simulink model "gm_CLKDIV_LED_basic"  (R2023a)
settings: Solver=VariableStepAuto  StartTime=0.0  StopTime=2  RelTol=1e-3
libraries: simulink x4
settings Model: Creator=criedl  LastModifiedBy=eduyilmet001
settings OptimizationCC: BlockReduction=off  ConditionallyExecuteInputs=off
settings DebuggingCC: ArtificialAlgebraicLoopMsg=none  InheritedTsInSrcMsg=none  UnconnectedInputMsg=warning  UnconnectedOutputMsg=warning  UnconnectedLineMsg=warning
settings ModelReferenceCC: EnableRefExpFcnMdlSchedulingChecks=on
settings RTWCC: DLArmComputeVersion=19.05

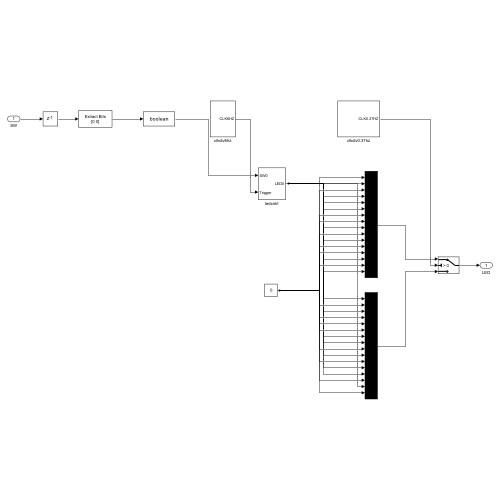
[thumbnail: Simulink's stored preview of the top-level diagram]
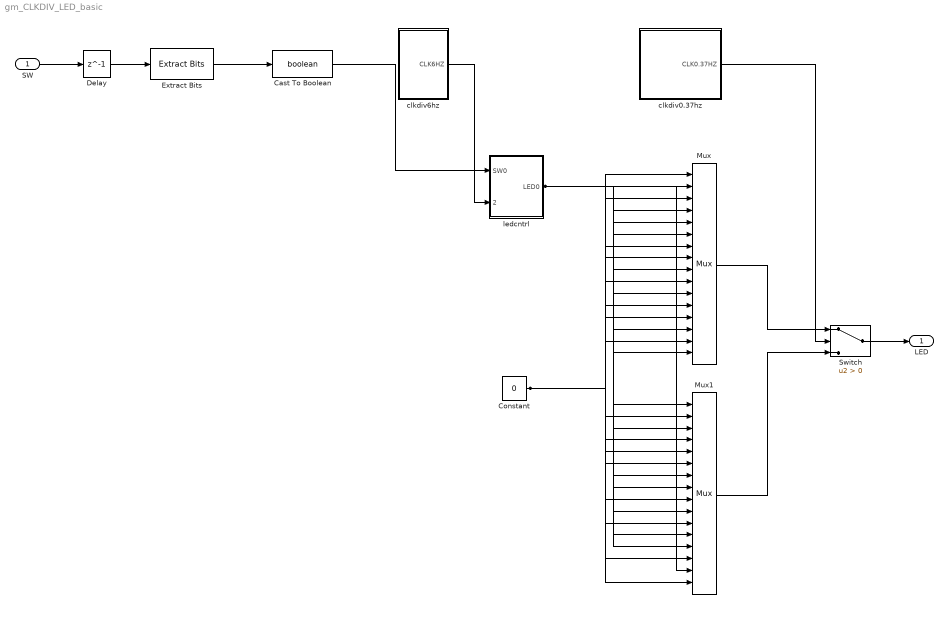
== system gm_CLKDIV_LED_basic ==
  SW : Inport  OutDataTypeStr=uint16  PortDimensions=1  SampleTime=1e-08
  Cast To Boolean : DataTypeConversion  OutDataTypeStr=boolean  SaturateOnIntegerOverflow=off  RndMeth=Floor
  Constant : Constant  Value=0  OutDataTypeStr=boolean
  Delay : Delay  DelayLength=1  InitialCondition=0
  Extract Bits : simulink/Logic and Bit Operations/Extract Bits  bitsToExtract=Range of bits  numBits=8  bitIdxRange=[0 0]  outScalingMode=Preserve fixed-point scaling
  Mux : Mux  Inputs=16
  Mux1 : Mux  Inputs=16
  Switch : Switch  Criteria=u2 > Threshold  SaturateOnIntegerOverflow=off  InputSameDT=off
  clkdiv0.37hz : Subsystem
  clkdiv6hz : Subsystem
  ledcntrl : Subsystem
  LED : Outport  SampleTime=1e-08  InitialOutput=0
  wires:
  SW/1 -> Delay/1
  Cast To Boolean/1 -> ledcntrl/1(SW0)
  Constant/1 -> Mux1/16, Mux1/14, Mux1/11, Mux1/9, Mux1/6, Mux1/5, Mux1/4, Mux1/2, Mux/15, Mux/13, Mux/12, Mux/10, Mux/8, Mux/7, Mux/3, Mux/1
  Delay/1 -> Extract Bits/1
  Extract Bits/1 -> Cast To Boolean/1
  Mux/1 -> Switch/1
  Mux1/1 -> Switch/3
  Switch/1 -> LED/1
  clkdiv0.37hz/1(CLK0.37HZ) -> Switch/2
  clkdiv6hz/1(CLK6HZ) -> ledcntrl/2(Trigger)
  ledcntrl/1(LED0) -> Mux1/15, Mux1/13, Mux1/12, Mux1/10, Mux1/8, Mux1/7, Mux1/3, Mux1/1, Mux/16, Mux/14, Mux/11, Mux/9, Mux/6, Mux/5, Mux/4, Mux/2

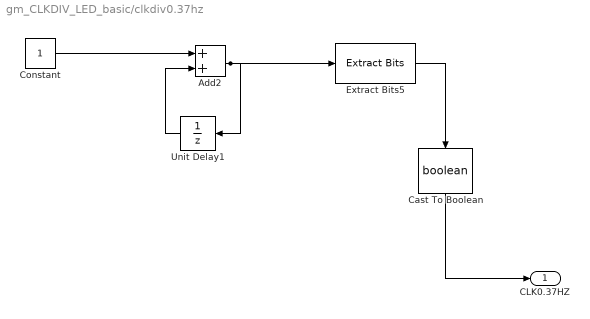
== system gm_CLKDIV_LED_basic/clkdiv0.37hz ==
  Add2 : Sum  AccumDataTypeStr=fixdt(0,29,0)  OutDataTypeStr=fixdt(0,29,0)
  Cast To Boolean : DataTypeConversion  OutDataTypeStr=boolean  SaturateOnIntegerOverflow=off  RndMeth=Floor
  Constant : Constant  OutDataTypeStr=boolean
  Extract Bits5 : simulink/Logic and Bit Operations/Extract Bits  bitsToExtract=Range of bits  numBits=8  bitIdxRange=[28 28]  outScalingMode=Preserve fixed-point scaling
  Unit Delay1 : UnitDelay  SampleTime=-1  HasFrameUpgradeWarning=on
  CLK0.37HZ : Outport  OutDataTypeStr=boolean  SampleTime=1e-08  InitialOutput=0
  wires:
  Add2/1 -> Extract Bits5/1, Unit Delay1/1
  Cast To Boolean/1 -> CLK0.37HZ/1
  Constant/1 -> Add2/1
  Extract Bits5/1 -> Cast To Boolean/1
  Unit Delay1/1 -> Add2/2

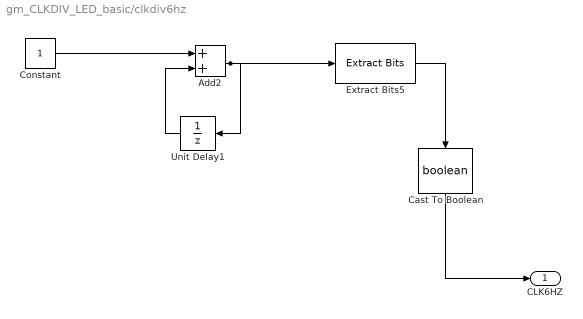
== system gm_CLKDIV_LED_basic/clkdiv6hz ==
  Add2 : Sum  AccumDataTypeStr=fixdt(0,24,0)  OutDataTypeStr=fixdt(0,24,0)
  Cast To Boolean : DataTypeConversion  OutDataTypeStr=boolean  SaturateOnIntegerOverflow=off  RndMeth=Floor
  Constant : Constant  OutDataTypeStr=boolean
  Extract Bits5 : simulink/Logic and Bit Operations/Extract Bits  bitsToExtract=Range of bits  numBits=8  bitIdxRange=[23 23]  outScalingMode=Preserve fixed-point scaling
  Unit Delay1 : UnitDelay  SampleTime=-1  HasFrameUpgradeWarning=on
  CLK6HZ : Outport  OutDataTypeStr=boolean  SampleTime=1e-08  InitialOutput=0
  wires:
  Add2/1 -> Extract Bits5/1, Unit Delay1/1
  Cast To Boolean/1 -> CLK6HZ/1
  Constant/1 -> Add2/1
  Extract Bits5/1 -> Cast To Boolean/1
  Unit Delay1/1 -> Add2/2

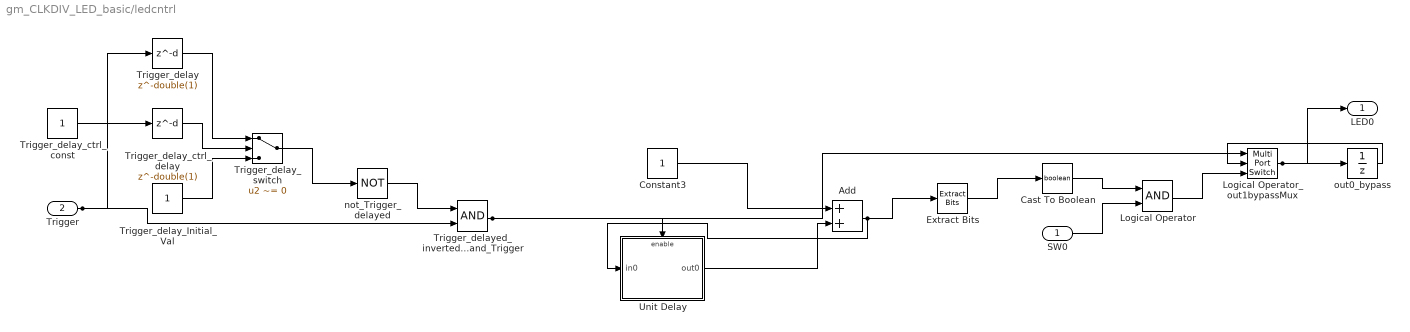
== system gm_CLKDIV_LED_basic/ledcntrl ==
  SW0 : Inport  OutDataTypeStr=boolean  PortDimensions=1  SampleTime=1e-08
  Trigger : Inport  Port=2  OutDataTypeStr=boolean  SampleTime=1e-08
  Add : Sum  AccumDataTypeStr=fixdt(0, 1, 0)  OutDataTypeStr=fixdt(0, 1, 0)  SampleTime=1e-08
  Cast To Boolean : DataTypeConversion  OutDataTypeStr=boolean  SampleTime=1e-08  SaturateOnIntegerOverflow=off  RndMeth=Floor
  Constant3 : Constant  OutDataTypeStr=boolean  SampleTime=1e-08
  Extract Bits : simulink/Logic and Bit Operations/Extract Bits  bitsToExtract=Range of bits  numBits=8  bitIdxRange=[0 0]  outScalingMode=Preserve fixed-point scaling
  Logical Operator : Logic  AllPortsSameDT=off  OutDataTypeStr=boolean  SampleTime=1e-08
  Logical Operator_out1bypassMux : MultiPortSwitch  DataPortOrder=Zero-based contiguous  Inputs=2  zeroidx=on  SampleTime=1e-08  SaturateOnIntegerOverflow=off  InputSameDT=off
  Trigger_delay : Delay  DelayLength=double(1)  InitialCondition=0
  Trigger_delay_Initial_Val : Constant  OutDataTypeStr=boolean  SampleTime=1e-08
  Trigger_delay_ctrl_const : Constant  OutDataTypeStr=boolean  SampleTime=1e-08
  Trigger_delay_ctrl_delay : Delay  DelayLength=double(1)  InitialCondition=0
  Trigger_delay_switch : Switch  Criteria=u2 ~= 0  Threshold=double(0)  OutDataTypeStr=boolean  SampleTime=1e-08  SaturateOnIntegerOverflow=off  InputSameDT=off
  Trigger_delayed_inverted_and_Trigger : Logic  AllPortsSameDT=off  OutDataTypeStr=boolean  SampleTime=1e-08
  Unit Delay : Subsystem
      settings: MinAlgLoopOccurrences=on
  not_Trigger_delayed : Logic  Operator=NOT  Inputs=1  AllPortsSameDT=off  OutDataTypeStr=boolean  SampleTime=1e-08
  out0_bypass : UnitDelay  SampleTime=1e-08
  LED0 : Outport  SampleTime=1e-08  InitialOutput=0
  wires:
  Trigger/1 -> Trigger_delayed_inverted_and_Trigger/2, Trigger_delay/1
  SW0/1 -> Logical Operator/2
  Logical Operator_out1bypassMux/1 -> LED0/1, out0_bypass/1
  Trigger_delay_switch/1 -> not_Trigger_delayed/1
  not_Trigger_delayed/1 -> Trigger_delayed_inverted_and_Trigger/1
  Trigger_delayed_inverted_and_Trigger/1 -> Logical Operator_out1bypassMux/1, Unit Delay/Enable
  Trigger_delay/1 -> Trigger_delay_switch/1
  Trigger_delay_Initial_Val/1 -> Trigger_delay_switch/3
  Trigger_delay_ctrl_const/1 -> Trigger_delay_ctrl_delay/1
  Trigger_delay_ctrl_delay/1 -> Trigger_delay_switch/2
  Add/1 -> Extract Bits/1, Unit Delay/1(in0)
  Cast To Boolean/1 -> Logical Operator/1
  Extract Bits/1 -> Cast To Boolean/1
  Constant3/1 -> Add/1
  Unit Delay/1(out0) -> Add/2
  Logical Operator/1 -> Logical Operator_out1bypassMux/3
  out0_bypass/1 -> Logical Operator_out1bypassMux/2

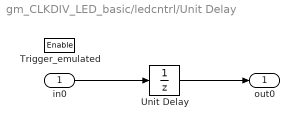
== system gm_CLKDIV_LED_basic/ledcntrl/Unit Delay ==
  in0 : Inport  OutDataTypeStr=fixdt(0,1,0,'DataTypeOverride', 'Off')  SampleTime=1e-08
  Trigger_emulated : EnablePort  OutDataTypeStr=boolean
  Unit Delay : UnitDelay  InitialCondition="fi(0,0,1,0,\"hex\",\"0\")"  SampleTime=1e-08
  out0 : Outport  OutDataTypeStr=fixdt(0, 1, 0)  SampleTime=1e-08  InitialOutput=0
  wires:
  Unit Delay/1 -> out0/1
  in0/1 -> Unit Delay/1
